simulink library "Susp_Components"  (R2026a)
settings: Solver=VariableStepAuto
undefined symbols (not defined in the file): Arm_to_Axle, clr_conn_links, clr_conn_rod, clr_link, clr_uaf, hp_in_f_ua, hp_out_f_ua, hp_shock_bot, hp_shock_botL, hp_shock_top, hp_shock_topL, hp_steerlink_out, hp_steerlink_outL, hp_upr_axle, hp_upr_axleL, hp_upr_drag, hp_upr_dragL, hp_wattsl_body, hp_wattsl_pivot, hp_wattsp_axle, hp_wattsu_body, hp_wattsu_pivot, hp_whl_ctr, hp_whl_ctrL, opc_conn_links, opc_conn_rod, opc_link, opc_uaf, radius_link, radius_uaf, size_conn_links, size_conn_rod, Susp, uaf_mass, upr_mass, Visual, wattsl_mass, wattsp_mass, wattsu_mass, X, Y, Z
libraries: sm_lib x32, Suspension_Utilities x10, Linkage_Shock x4, nesl_utility x3, $bdroot x2, simulink_extras x1
(part 1 of 2)
Description:
  | Component of Simscape Vehicle Templates Library
  | 
  | Copyright 2018-2025 The MathWorks, Inc.
settings Model: Creator=mwalker  LastModifiedBy=smiller

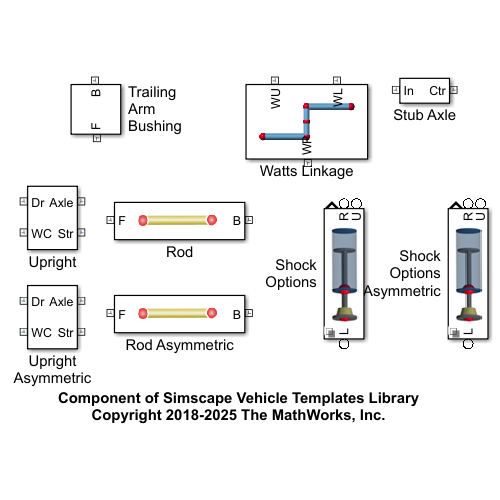
[thumbnail: Simulink's stored preview of the top-level diagram]
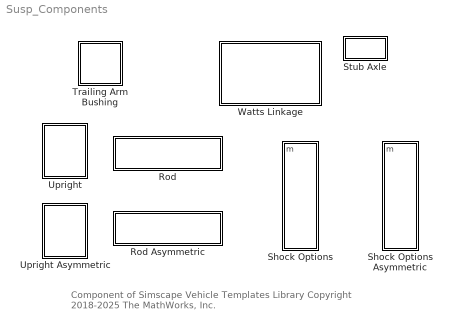
== system Susp_Components ==
  note: Component of Simscape Vehicle Templates Library
      | Copyright 2018-2025 The MathWorks, Inc.
  Rod : Subsystem  VariantControl=Steer  mask(Arm){popup_leftRight=Left, hp_in=hp_in_f_ua, hp_out=hp_out_f_ua, rod_mass=uaf_mass, clr_conn_rod=clr_conn_links, opc_conn_rod=opc_conn_links, size_conn_rod=size_conn_links, clr_rod=clr_uaf, opc_rod=opc_uaf, radius_rod=radius_uaf}
      mask prompts: popup_leftRight "Left/Right"; hp_in "HP B [xyz] (m)"; hp_out "HP F [xyz] (m)"; rod_mass "Mass (kg)"
      mask help: Rigid arm with two connection points.
      mask init:
      | if(popup_leftRight == 1)
      |     rhs_rod = 1;
      | elseif(popup_leftRight == 2)
      |     rhs_rod = -1;
      | end
      mask TypeOptions popup_leftRight: Left | Right
      mask TypeOptions rod_mass: Rod/Mass
      mask TypeOptions clr_conn_rod:
      | Vis
      | HP A/GraphicDiffuseColor | Vis
      | HP B/GraphicDiffuseColor
      mask TypeOptions opc_conn_rod:
      | Vis
      | HP A/GraphicOpacity | Vis
      | HP B/GraphicOpacity
      mask TypeOptions clr_rod: Rod/clr_solid
      mask TypeOptions opc_rod: Rod/opc_solid
      mask TypeOptions radius_rod: Rod/rad_solid
      mask DialogControl cont_rod Prompt: Rod
      mask DialogControl grp_rod Prompt: Rod
      mask DialogControl cont_vis_rod Prompt: Visualization
      mask DialogControl text_clr_rod Prompt: Color [RGB]
      mask DialogControl text_opc_rod Prompt: Opac. (0-1)
      mask DialogControl text_size_rod Prompt: Size (m)
      mask DialogControl text_conn_rod Prompt: Connections
      mask DialogControl text_rod_rod Prompt: Rod
      mask Display: image('sm_car_vehicle_linkage_link_IMAGE.png');
  Rod Asymmetric : Subsystem  VariantControl=Steer  mask(Arm){hp_in=hp_in_f_ua, hp_out=hp_out_f_ua, rod_mass=uaf_mass, clr_conn_rod=clr_conn_links, opc_conn_rod=opc_conn_links, size_conn_rod=size_conn_links, clr_rod=clr_uaf, opc_rod=opc_uaf, radius_rod=radius_uaf}
      mask prompts: hp_in "HP B [xyz] (m)"; hp_out "HP F [xyz] (m)"; rod_mass "Mass (kg)"
      mask help: Rigid arm with two connection points.
      mask TypeOptions rod_mass: Rod/Mass
      mask TypeOptions clr_conn_rod:
      | Vis
      | HP A/GraphicDiffuseColor | Vis
      | HP B/GraphicDiffuseColor
      mask TypeOptions opc_conn_rod:
      | Vis
      | HP A/GraphicOpacity | Vis
      | HP B/GraphicOpacity
      mask TypeOptions clr_rod: Rod/clr_solid
      mask TypeOptions opc_rod: Rod/opc_solid
      mask TypeOptions radius_rod: Rod/rad_solid
      mask DialogControl cont_rod Prompt: Rod
      mask DialogControl grp_rod Prompt: Rod
      mask DialogControl cont_vis_rod Prompt: Visualization
      mask DialogControl text_clr_rod Prompt: Color [RGB]
      mask DialogControl text_opc_rod Prompt: Opac. (0-1)
      mask DialogControl text_size_rod Prompt: Size (m)
      mask DialogControl text_conn_rod Prompt: Connections
      mask DialogControl text_rod_rod Prompt: Rod
      mask Display: image('sm_car_vehicle_linkage_link_IMAGE.png');
  Shock Options : Subsystem  Variant=on  VariantControlMode=label  VariantControl=ShockL  LabelModeActiveChoice=CylUpAttCtr  mask{popup_leftRight=Left, VariantLabel='CylUpAttCtr'}
      mask prompts: popup_leftRight "Left/Right"; VariantLabel "Variant Label"
      mask init:
      | curblk = gcb;
      | 
      | % Set variant for this block 
      | set_param(curblk,'LabelModeActiveChoice',VariantLabel);
      | 
      | if(popup_leftRight == 1)
      |     rhs_rod = 1;
      | elseif(popup_leftRight == 2)
      |     rhs_rod = -1;
      | end
      mask TypeOptions popup_leftRight: Left | Right
  Shock Options Asymmetric : Subsystem  Variant=on  VariantControlMode=label  VariantControl=ShockL  LabelModeActiveChoice=CylUpAttCtr  mask{hp_shock_top=hp_shock_topL, hp_shock_bot=hp_shock_botL, VariantLabel='CylUpAttCtr'}
      mask prompts: hp_shock_top "Spring Top [xyz] (m)"; hp_shock_bot "Spring Bottom [xyz] (m)"; VariantLabel "Variant Label"
      mask init:
      | curblk = gcb;
      | 
      | % Set variant for this block 
      | set_param(curblk,'LabelModeActiveChoice',VariantLabel);
  Stub Axle : Subsystem  mask{popup_leftRight=Left, stub_axle_len=Susp.AxleTA4Watts.Axle.xAxle.Value, stub_axle_mass=Susp.AxleTA4Watts.StubAxle.m.Value, clr_stub_axle=Visual.Axle.clr, opc_stub_axle=Visual.part.opc, rad_stub_axle=Visual.Axle.rad}
      mask prompts: popup_leftRight "Left/Right"; stub_axle_len "Stub Axle Length (m)"; stub_axle_mass "Stub Axle Mass (kg)"; clr_stub_axle "Color [RGB]"; opc_stub_axle "Opacity (0-1)"; rad_stub_axle "Stub Axle Radius (m)"
      mask init:
      | if(popup_leftRight == 1)
      |     rhs_rod = 1;
      | elseif(popup_leftRight == 2)
      |     rhs_rod = -1;
      | end
      mask TypeOptions popup_leftRight: Left | Right
      mask TypeOptions stub_axle_mass: Axle/Mass
      mask TypeOptions clr_stub_axle: Axle/GraphicDiffuseColor
      mask TypeOptions opc_stub_axle: Axle/GraphicOpacity
      mask TypeOptions rad_stub_axle: Axle/CylinderRadius
      mask DialogControl cont_vis Prompt: Visualization
  Trailing Arm Bushing : Subsystem  mask{Arm_to_Axle=Arm_to_Axle}
      mask prompts: Arm_to_Axle "Arm to Axle (structure)"
  Upright : Subsystem  mask(Upright, Three Connections){popup_leftRight=Left, clr_conn_rod=Visual.hp.clr, opc_conn_rod=Visual.hp.opc, size_conn_rod=Visual.hp.rad, clr_upr=Visual.Upright.clr, opc_upr=Visual.part.opc, rad_upr=Visual.Upright.rad}
      mask prompts: popup_leftRight "Left/Right"; clr_conn_rod "Connections Color [R G B] (0-1)"; opc_conn_rod "Connections Opacity (0-1)"; size_conn_rod "Connections Radius (m)"; clr_upr "Link Color [R G B] (0-1)"; opc_upr "Link Opacity (0-1)"; rad_upr "Link Radius (0-1)"
      mask help: Models an upright with connections to the axle along the kingpin axis (Axle), wheel center (WC), drag link (Dr), and steering link (Str).
      mask init:
      | if(popup_leftRight == 1)
      |     rhs_upr = 1;
      | elseif(popup_leftRight == 2)
      |     rhs_upr = -1;
      | end
      | rhs_hp = [1 rhs_upr 1];
      mask TypeOptions popup_leftRight: Left | Right
      mask DialogControl cont_vis Prompt: Visualization
  Upright Asymmetric : Subsystem  mask(Upright, Three Connections){hp_upr_axle=hp_upr_axleL, hp_whl_ctr=hp_whl_ctrL, hp_upr_drag=hp_upr_dragL, hp_steerlink_out=hp_steerlink_outL, clr_conn_rod=Visual.hp.clr, opc_conn_rod=Visual.hp.opc, size_conn_rod=Visual.hp.rad, clr_upr=Visual.Upright.clr, opc_upr=Visual.part.opc, rad_upr=Visual.Upright.rad}
      mask prompts: hp_upr_axle "Hardpoint Upright Axle [xyz] (m)"; hp_whl_ctr "Hardpoint Wheel Center [xyz] (m)"; hp_upr_drag "Hardpoint Drag Link [xyz] (m)"; hp_steerlink_out "Hardpoint Steer Link  [xyz] (m)"; clr_conn_rod "Connections Color [R G B] (0-1)"; opc_conn_rod "Connections Opacity (0-1)"; size_conn_rod "Connections Radius (m)"; clr_upr "Link Color [R G B] (0-1)"; opc_upr "Link Opacity (0-1)"; rad_upr "Link Radius (0-1)"
      mask help: Models an upright with connections to the axle along the kingpin axis (Axle), wheel center (WC), drag link (Dr), and steering link (Str).
      mask TypeOptions hp_upr_axle: Drag/hp_b | Steer/hp_b | Upright/hp_b
      mask TypeOptions hp_whl_ctr: Upright/hp_f
      mask TypeOptions hp_upr_drag: Drag/hp_f
      mask TypeOptions hp_steerlink_out: Steer/hp_f
      mask DialogControl cont_vis Prompt: Visualization
  Watts Linkage : Subsystem  mask(Watts Linkage){hp_wattsu_body=hp_wattsu_body, hp_wattsl_body=hp_wattsl_body, hp_wattsu_pivot=hp_wattsu_pivot, hp_wattsl_pivot=hp_wattsl_pivot, hp_wattsp_axle=hp_wattsp_axle, wattsu_mass=wattsu_mass, wattsl_mass=wattsl_mass, wattsp_mass=wattsp_mass, clr_conn_rod=clr_conn_rod, opc_conn_rod=opc_conn_rod, size_conn_rod=size_conn_rod, clr_link=clr_link, opc_link=opc_link, radius_link=radius_link}
      mask prompts: hp_wattsu_body "Watts Link Upper Body [xyz] (m)"; hp_wattsl_body "Watts Link Lower Body [xyz] (m)"; hp_wattsu_pivot "Watts Link Upper to Pivot [xyz] (m)"; hp_wattsl_pivot "Watts Link Lower to Pivot [xyz] (m)"; hp_wattsp_axle "Watts Link Pivot to Axle [xyz] (m)"; wattsu_mass "Watts Link Upper Mass (kg)"; wattsl_mass "Watts Link Lower Mass (kg)"; wattsp_mass "Watts Link Pivot Mass (kg)"
      mask help: Models a Watts linkage with upper, lower, and pivot links.
      mask TypeOptions hp_wattsu_body:
      | Watts Link
      | Upper/hp_in
      mask TypeOptions hp_wattsl_body:
      | Watts Link
      | Lower/hp_in
      mask TypeOptions hp_wattsu_pivot:
      | Watts Link
      | Pivot/hp_b | Watts Link
      | Upper/hp_out
      mask TypeOptions hp_wattsl_pivot:
      | Watts Link
      | Lower/hp_out | Watts Link
      | Pivot/hp_f
      mask TypeOptions hp_wattsp_axle:
      | Watts Link
      | Pivot/hp_piv
      mask TypeOptions wattsu_mass:
      | Watts Link
      | Upper/rod_mass
      mask TypeOptions wattsl_mass:
      | Watts Link
      | Lower/rod_mass
      mask TypeOptions wattsp_mass:
      | Watts Link
      | Pivot/rod_mass
      mask TypeOptions clr_conn_rod:
      | Watts Link
      | Lower/clr_conn_rod | Watts Link
      | Pivot/clr_conn_rod | Watts Link
      | Upper/clr_conn_rod
      mask TypeOptions opc_conn_rod:
      | Watts Link
      | Lower/opc_conn_rod | Watts Link
      | Pivot/opc_conn_rod | Watts Link
      | Upper/opc_conn_rod
      mask TypeOptions size_conn_rod:
      | Watts Link
      | Lower/size_conn_rod | Watts Link
      | Pivot/size_conn_rod | Watts Link
      | Upper/size_conn_rod
      mask TypeOptions clr_link:
      | Watts Link
      | Lower/clr_rod | Watts Link
      | Pivot/clr_rod | Watts Link
      | Upper/clr_rod
      mask TypeOptions opc_link:
      | Watts Link
      | Lower/opc_rod | Watts Link
      | Pivot/opc_rod | Watts Link
      | Upper/opc_rod
      mask TypeOptions radius_link:
      | Watts Link
      | Lower/radius_rod | Watts Link
      | Pivot/radius_rod | Watts Link
      | Upper/radius_rod
      mask DialogControl cont_hp Prompt: Hardpoints
      mask DialogControl cont_parts Prompt: Parts
      mask DialogControl cont_parts_vis Prompt: Visualization
      mask DialogControl text_vis_clr Prompt: Color [RGB]
      mask DialogControl text_vis_opc Prompt: Opac. (0-1)
      mask DialogControl text_vis_size Prompt: Size (m)
      mask DialogControl text_vis_conn Prompt: Connections
      mask DialogControl text_vis_links Prompt: Links
      mask Display: image('sm_car_vehicle_susp_wattslinkage_image.png');

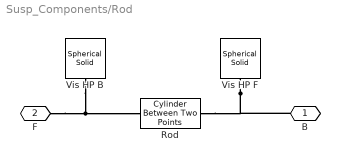
== system Susp_Components/Rod ==
  Rod : Suspension_Utilities/Cylinder Between Two Points  hp_b=hp_in.*[1 rhs_rod 1]  hp_f=hp_out.*[1 rhs_rod 1]  Mass=rod_mass  clr_solid=clr_rod  opc_solid=opc_rod  rad_solid=radius_rod
  Vis HP B : sm_lib/Body Elements/Spherical Solid  SphereRadius=size_conn_rod  SphereRadiusUnits=m  ExportEntireGeometry=off  InertiaType=CalculateFromGeometry  BasedOnType=Density  Density=0  DensityUnits=kg/m^3  Mass=1  MassUnits=kg  CenterOfMass=[0 0 0]  CenterOfMassUnits=m  MomentsOfInertia=[1 1 1]  MomentsOfInertiaUnits=kg*m^2  ProductsOfInertia=[0 0 0]  ProductsOfInertiaUnits=kg*m^2  GraphicType=FromGeometry  MarkerShape=Sphere  MarkerSize=10  GraphicVisPropType=SimpleVisualProperties  GraphicDiffuseColor=clr_conn_rod  GraphicOpacity=opc_conn_rod  GraphicSpecularColor=[0.5 0.5 0.5 1.0]  GraphicAmbientColor=[0.15 0.15 0.15 1.0]  GraphicEmissiveColor=[0.0 0.0 0.0 1.0]  GraphicShininess=75  DoExposeReferenceFrame=on  SerializedFrames=<Frames/>
  Vis HP F : sm_lib/Body Elements/Spherical Solid  SphereRadius=size_conn_rod  SphereRadiusUnits=m  ExportEntireGeometry=off  InertiaType=CalculateFromGeometry  BasedOnType=Density  Density=0  DensityUnits=kg/m^3  Mass=1  MassUnits=kg  CenterOfMass=[0 0 0]  CenterOfMassUnits=m  MomentsOfInertia=[1 1 1]  MomentsOfInertiaUnits=kg*m^2  ProductsOfInertia=[0 0 0]  ProductsOfInertiaUnits=kg*m^2  GraphicType=FromGeometry  MarkerShape=Sphere  MarkerSize=10  GraphicVisPropType=SimpleVisualProperties  GraphicDiffuseColor=clr_conn_rod  GraphicOpacity=opc_conn_rod  GraphicSpecularColor=[0.5 0.5 0.5 1.0]  GraphicAmbientColor=[0.15 0.15 0.15 1.0]  GraphicEmissiveColor=[0.0 0.0 0.0 1.0]  GraphicShininess=75  DoExposeReferenceFrame=on  SerializedFrames=<Frames/>
  B : PMIOPort  Side=Right
  F : PMIOPort  Port=2  Side=Left
  connections:
  Vis HP F/RConn1 -- B/RConn1 -- Rod/LConn1
  F/RConn1 -- Rod/RConn1 -- Vis HP B/RConn1

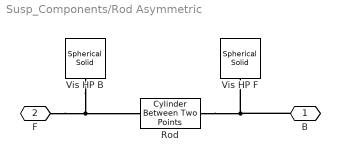
== system Susp_Components/Rod Asymmetric ==
  Rod : Suspension_Utilities/Cylinder Between Two Points  hp_b=hp_in  hp_f=hp_out  Mass=rod_mass  clr_solid=clr_rod  opc_solid=opc_rod  rad_solid=radius_rod
  Vis HP B : sm_lib/Body Elements/Spherical Solid  SphereRadius=size_conn_rod  SphereRadiusUnits=m  ExportEntireGeometry=off  InertiaType=CalculateFromGeometry  BasedOnType=Density  Density=0  DensityUnits=kg/m^3  Mass=1  MassUnits=kg  CenterOfMass=[0 0 0]  CenterOfMassUnits=m  MomentsOfInertia=[1 1 1]  MomentsOfInertiaUnits=kg*m^2  ProductsOfInertia=[0 0 0]  ProductsOfInertiaUnits=kg*m^2  GraphicType=FromGeometry  MarkerShape=Sphere  MarkerSize=10  GraphicVisPropType=SimpleVisualProperties  GraphicDiffuseColor=clr_conn_rod  GraphicOpacity=opc_conn_rod  GraphicSpecularColor=[0.5 0.5 0.5 1.0]  GraphicAmbientColor=[0.15 0.15 0.15 1.0]  GraphicEmissiveColor=[0.0 0.0 0.0 1.0]  GraphicShininess=75  DoExposeReferenceFrame=on  SerializedFrames=<Frames/>
  Vis HP F : sm_lib/Body Elements/Spherical Solid  SphereRadius=size_conn_rod  SphereRadiusUnits=m  ExportEntireGeometry=off  InertiaType=CalculateFromGeometry  BasedOnType=Density  Density=0  DensityUnits=kg/m^3  Mass=1  MassUnits=kg  CenterOfMass=[0 0 0]  CenterOfMassUnits=m  MomentsOfInertia=[1 1 1]  MomentsOfInertiaUnits=kg*m^2  ProductsOfInertia=[0 0 0]  ProductsOfInertiaUnits=kg*m^2  GraphicType=FromGeometry  MarkerShape=Sphere  MarkerSize=10  GraphicVisPropType=SimpleVisualProperties  GraphicDiffuseColor=clr_conn_rod  GraphicOpacity=opc_conn_rod  GraphicSpecularColor=[0.5 0.5 0.5 1.0]  GraphicAmbientColor=[0.15 0.15 0.15 1.0]  GraphicEmissiveColor=[0.0 0.0 0.0 1.0]  GraphicShininess=75  DoExposeReferenceFrame=on  SerializedFrames=<Frames/>
  B : PMIOPort  Side=Right
  F : PMIOPort  Port=2  Side=Left
  connections:
  Vis HP B/RConn1 -- Rod/RConn1 -- F/RConn1
  Rod/LConn1 -- B/RConn1 -- Vis HP F/RConn1

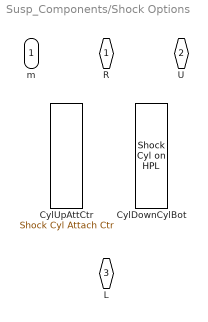
== system Susp_Components/Shock Options ==
  CylDownCylBot : Linkage_Shock/Shock Cyl on HPL  VariantControl=CylDownCylBot  shock_pist_mass=piston_mass  shock_cyl_mass=cyl_mass  hp_spr_top=hp_shock_top.*[1 rhs_rod 1]  hp_spr_bot=hp_shock_bot.*[1 rhs_rod 1]  up_lim_bumpstop=shock_xmax  low_lim_bumpstop=shock_xmin  clr_conn_shock=Visual.hp.clr  opc_conn_shock=Visual.hp.opc  size_conn_shock=Visual.hp.rad  clr_shock_cyl=Visual.clr.blue  opc_shock_cyl=Visual.part.opc  radius_shock_cyl=0.05  clr_shock_piston=Visual.clr.gray  opc_shock_piston=Visual.part.opc  clr_shock_bumpstop=Visual.clr.yellowpale  opc_shock_bumpstop=Visual.part.opc  deadvol_len_shock_cyl=Visual.Shock.dead_length  piston_len_shock=Visual.Shock.piston.len  cyl_cap_len_shock=Visual.Shock.cap.len  bumpstop_len_shock=Visual.Shock.bumpstop.len
  CylUpAttCtr : Linkage_Shock/Shock Cyl Attach Ctr  VariantControl=CylUpAttCtr  shock_pist_mass=piston_mass  shock_cyl_mass=cyl_mass  hp_spr_top=hp_shock_top.*[1 rhs_rod 1]  hp_spr_bot=hp_shock_bot.*[1 rhs_rod 1]  up_lim_bumpstop=shock_xmax  low_lim_bumpstop=shock_xmin  clr_conn_shock=Visual.hp.clr  opc_conn_shock=Visual.hp.opc  size_conn_shock=Visual.hp.rad  clr_shock_cyl=Visual.clr.blue  opc_shock_cyl=Visual.part.opc  radius_shock_cyl=0.05  clr_shock_piston=Visual.clr.gray  opc_shock_piston=Visual.part.opc  clr_shock_bumpstop=Visual.clr.yellowpale  opc_shock_bumpstop=Visual.part.opc  deadvol_len_shock_cyl=Visual.Shock.dead_length  piston_len_shock=Visual.Shock.piston.len  cyl_cap_len_shock=Visual.Shock.cap.len  bumpstop_len_shock=Visual.Shock.bumpstop.len
  R : PMIOPort  Side=Right
  U : PMIOPort  Port=2  Side=Right
  L : PMIOPort  Port=3  Side=Left
  m : Outport

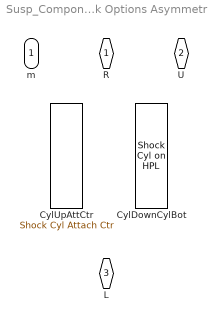
== system Susp_Components/Shock Options Asymmetric ==
  CylDownCylBot : Linkage_Shock/Shock Cyl on HPL  VariantControl=CylDownCylBot  shock_pist_mass=piston_mass  shock_cyl_mass=cyl_mass  hp_spr_top=hp_shock_top  hp_spr_bot=hp_shock_bot  up_lim_bumpstop=shock_xmax  low_lim_bumpstop=shock_xmin  clr_conn_shock=Visual.hp.clr  opc_conn_shock=Visual.hp.opc  size_conn_shock=Visual.hp.rad  clr_shock_cyl=Visual.clr.blue  opc_shock_cyl=Visual.part.opc  radius_shock_cyl=0.05  clr_shock_piston=Visual.clr.gray  opc_shock_piston=Visual.part.opc  clr_shock_bumpstop=Visual.clr.yellowpale  opc_shock_bumpstop=Visual.part.opc  deadvol_len_shock_cyl=Visual.Shock.dead_length  piston_len_shock=Visual.Shock.piston.len  cyl_cap_len_shock=Visual.Shock.cap.len  bumpstop_len_shock=Visual.Shock.bumpstop.len
  CylUpAttCtr : Linkage_Shock/Shock Cyl Attach Ctr  VariantControl=CylUpAttCtr  shock_pist_mass=piston_mass  shock_cyl_mass=cyl_mass  hp_spr_top=hp_shock_top  hp_spr_bot=hp_shock_bot  up_lim_bumpstop=shock_xmax  low_lim_bumpstop=shock_xmin  clr_conn_shock=Visual.hp.clr  opc_conn_shock=Visual.hp.opc  size_conn_shock=Visual.hp.rad  clr_shock_cyl=Visual.clr.blue  opc_shock_cyl=Visual.part.opc  radius_shock_cyl=0.05  clr_shock_piston=Visual.clr.gray  opc_shock_piston=Visual.part.opc  clr_shock_bumpstop=Visual.clr.yellowpale  opc_shock_bumpstop=Visual.part.opc  deadvol_len_shock_cyl=Visual.Shock.dead_length  piston_len_shock=Visual.Shock.piston.len  cyl_cap_len_shock=Visual.Shock.cap.len  bumpstop_len_shock=Visual.Shock.bumpstop.len
  R : PMIOPort  Side=Right
  U : PMIOPort  Port=2  Side=Right
  L : PMIOPort  Port=3  Side=Left
  m : Outport

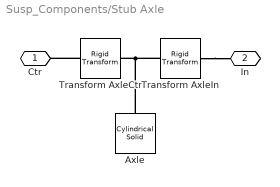
== system Susp_Components/Stub Axle ==
  Axle : sm_lib/Body Elements/Cylindrical Solid  CylinderRadius=rad_stub_axle  CylinderRadiusUnits=m  CylinderLength=stub_axle_len  CylinderLengthUnits=m  ExportEntireGeometry=off  InertiaType=CalculateFromGeometry  BasedOnType=Mass  Density=7000  DensityUnits=kg/m^3  Mass=stub_axle_mass  MassUnits=kg  CenterOfMass=[0 0 0]  CenterOfMassUnits=m  MomentsOfInertia=[1 1 1]  MomentsOfInertiaUnits=kg*m^2  ProductsOfInertia=[0 0 0]  ProductsOfInertiaUnits=kg*m^2  GraphicType=FromGeometry  MarkerShape=Sphere  MarkerSize=10  GraphicVisPropType=SimpleVisualProperties  GraphicDiffuseColor=clr_stub_axle  GraphicOpacity=opc_stub_axle  GraphicSpecularColor=[0.5 0.5 0.5 1.0]  GraphicAmbientColor=[0.15 0.15 0.15 1.0]  GraphicEmissiveColor=[0.0 0.0 0.0 1.0]  GraphicShininess=75  DoExposeReferenceFrame=on  SerializedFrames=<Frames/>
  Transform AxleCtr : sm_lib/Frames and Transforms/Rigid Transform  RotationMethod=None  FollAlignAxisA=+X  BaseAlignAxisA=+Y  FollAlignAxisB=+Y  BaseAlignAxisB=+Z  RotationStandardAxis=+Z  RotationAngle=0  RotationAngleUnits=deg  RotationArbitraryAxis=[0 0 1]  RotationSequenceAxes=FollowerAxes  RotationSequence=XYX  RotationSequenceAngles=[0 0 0]  RotationSequenceAnglesUnits=deg  RotationMatrix=[1 0 0; 0 1 0; 0 0 1]  Quaternion=[1 0 0 0]  TranslationMethod=StandardAxis  TranslationCartesianOffset=[0 0 0]  TranslationCartesianOffsetUnits=m  TranslationStandardAxis=-Z  TranslationStandardOffset=rhs_rod*stub_axle_len/2  TranslationStandardOffsetUnits=m  TranslationROffset=0  TranslationROffsetUnits=m  TranslationThetaOffset=0  TranslationThetaOffsetUnits=deg  TranslationZOffset=0  TranslationZOffsetUnits=m
  Transform AxleIn : sm_lib/Frames and Transforms/Rigid Transform  RotationMethod=None  FollAlignAxisA=+X  BaseAlignAxisA=+Y  FollAlignAxisB=+Y  BaseAlignAxisB=+Z  RotationStandardAxis=+Z  RotationAngle=0  RotationAngleUnits=deg  RotationArbitraryAxis=[0 0 1]  RotationSequenceAxes=FollowerAxes  RotationSequence=XYX  RotationSequenceAngles=[0 0 0]  RotationSequenceAnglesUnits=deg  RotationMatrix=[1 0 0; 0 1 0; 0 0 1]  Quaternion=[1 0 0 0]  TranslationMethod=StandardAxis  TranslationCartesianOffset=[0 0 0]  TranslationCartesianOffsetUnits=m  TranslationStandardAxis=-Z  TranslationStandardOffset=rhs_rod*stub_axle_len/2  TranslationStandardOffsetUnits=m  TranslationROffset=0  TranslationROffsetUnits=m  TranslationThetaOffset=0  TranslationThetaOffsetUnits=deg  TranslationZOffset=0  TranslationZOffsetUnits=m
  Ctr : PMIOPort  Side=Left
  In : PMIOPort  Port=2  Side=Right
  connections:
  Transform AxleIn/RConn1 -- In/RConn1
  Transform AxleCtr/LConn1 -- Ctr/RConn1
  Transform AxleIn/LConn1 -- Transform AxleCtr/RConn1 -- Axle/RConn1

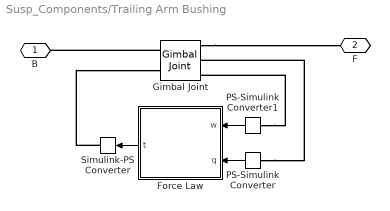
== system Susp_Components/Trailing Arm Bushing ==
  Force Law : Subsystem  mask{nLinear=Arm_to_Axle.Damping.nLinear.Value, nCubic=Arm_to_Axle.Damping.nCubic.Value, qStiffness=Arm_to_Axle.Stiffness.q.Value, trqStiffness=Arm_to_Axle.Stiffness.trq.Value, wFriction=Arm_to_Axle.Friction.w.Value, trqFriction=Arm_to_Axle.Friction.trq.Value}
      mask prompts: nLinear "Linear Gain"; nCubic "Cubic Gain"; qStiffness "Angle (rad)"; trqStiffness "Torque (N*m)"; wFriction "Rotational Velocity (rad/s)"; trqFriction "Torque (N*m)"
      mask TypeOptions nLinear: Gain Linear Term/Gain
      mask TypeOptions nCubic: Gain Exp Term/Gain
      mask TypeOptions qStiffness: Torsional Stiffness/BreakpointsForDimension1
      mask TypeOptions trqStiffness: Torsional Stiffness/Table
      mask TypeOptions wFriction: Friction/BreakpointsForDimension1
      mask TypeOptions trqFriction: Friction/Table
      mask DialogControl grpStiffness Prompt: Stiffness
      mask DialogControl grpFriction Prompt: Friction
      mask DialogControl grpDamping Prompt: Damping
  Gimbal Joint : sm_lib/Joints/Gimbal Joint  JointMode=Normal  CompositeWrenchDir=FollowerOnBase  CompositeWrenchFrame=BaseFrame  SenseConstraintForce=off  SenseConstraintTorque=off  SenseTotalForce=off  SenseTotalTorque=off  RxPositionTargetSpecify=on  RxPositionTargetPriority=Low  RxPositionTargetValue=0  RxPositionTargetValueUnits=deg  RxVelocityTargetSpecify=off  RxVelocityTargetPriority=High  RxVelocityTargetValue=0  RxVelocityTargetValueUnits=deg/s  RxEquilibriumPosition=0  RxEquilibriumPositionUnits=deg  RxSpringStiffness=0  RxSpringStiffnessUnits=N*m/deg  RxDampingCoefficient=0  RxDampingCoefficientUnits=N*m/(deg/s)  RxLowerLimitSpecify=off  RxLowerLimitBound=-90  RxLowerLimitBoundUnits=deg  RxLowerLimitStiffness=1e4  RxLowerLimitStiffnessUnits=N*m/deg  RxLowerLimitDamping=10  RxLowerLimitDampingUnits=N*m/(deg/s)  RxLowerLimitTransitionRegionWidth=0.1  RxLowerLimitTransitionRegionWidthUnits=deg  RxUpperLimitSpecify=off  RxUpperLimitBound=90  RxUpperLimitBoundUnits=deg  RxUpperLimitStiffness=1e4  RxUpperLimitStiffnessUnits=N*m/deg  RxUpperLimitDamping=10  RxUpperLimitDampingUnits=N*m/(deg/s)  RxUpperLimitTransitionRegionWidth=0.1  RxUpperLimitTransitionRegionWidthUnits=deg  RxTorqueActuationMode=NoTorque  RxMotionActuationMode=ComputedMotion  RxSensePosition=off  RxSenseVelocity=off  RxSenseAcceleration=off  RxSenseTorqueForce=off  RxSenseLowerLimitTorqueForce=off  RxSenseUpperLimitTorqueForce=off  RyPositionTargetSpecify=on  RyPositionTargetPriority=Low  RyPositionTargetValue=0  RyPositionTargetValueUnits=deg  RyVelocityTargetSpecify=off  RyVelocityTargetPriority=High  RyVelocityTargetValue=0  RyVelocityTargetValueUnits=deg/s  RyEquilibriumPosition=0  RyEquilibriumPositionUnits=deg  RySpringStiffness=0  RySpringStiffnessUnits=N*m/deg  RyDampingCoefficient=0  RyDampingCoefficientUnits=N*m/(deg/s)  RyLowerLimitSpecify=off  RyLowerLimitBound=-90  RyLowerLimitBoundUnits=deg  RyLowerLimitStiffness=1e4  RyLowerLimitStiffnessUnits=N*m/deg  RyLowerLimitDamping=10  RyLowerLimitDampingUnits=N*m/(deg/s)  RyLowerLimitTransitionRegionWidth=0.1  RyLowerLimitTransitionRegionWidthUnits=deg  RyUpperLimitSpecify=off  RyUpperLimitBound=90  RyUpperLimitBoundUnits=deg  RyUpperLimitStiffness=1e4  RyUpperLimitStiffnessUnits=N*m/deg  RyUpperLimitDamping=10  RyUpperLimitDampingUnits=N*m/(deg/s)  RyUpperLimitTransitionRegionWidth=0.1  RyUpperLimitTransitionRegionWidthUnits=deg  RyTorqueActuationMode=InputTorque  RyMotionActuationMode=ComputedMotion  RySensePosition=on  RySenseVelocity=on  RySenseAcceleration=off  RySenseTorqueForce=off  RySenseLowerLimitTorqueForce=off  RySenseUpperLimitTorqueForce=off  RzPositionTargetSpecify=off  RzPositionTargetPriority=High  RzPositionTargetValue=0  RzPositionTargetValueUnits=deg  RzVelocityTargetSpecify=off  RzVelocityTargetPriority=High  RzVelocityTargetValue=0  RzVelocityTargetValueUnits=deg/s  RzEquilibriumPosition=0  RzEquilibriumPositionUnits=deg  RzSpringStiffness=0  RzSpringStiffnessUnits=N*m/deg  RzDampingCoefficient=0  RzDampingCoefficientUnits=N*m/(deg/s)  RzLowerLimitSpecify=off  RzLowerLimitBound=-90  RzLowerLimitBoundUnits=deg  RzLowerLimitStiffness=1e4  RzLowerLimitStiffnessUnits=N*m/deg  RzLowerLimitDamping=10  RzLowerLimitDampingUnits=N*m/(deg/s)  RzLowerLimitTransitionRegionWidth=0.1  RzLowerLimitTransitionRegionWidthUnits=deg  RzUpperLimitSpecify=off  RzUpperLimitBound=90  RzUpperLimitBoundUnits=deg  RzUpperLimitStiffness=1e4  RzUpperLimitStiffnessUnits=N*m/deg  RzUpperLimitDamping=10  RzUpperLimitDampingUnits=N*m/(deg/s)  RzUpperLimitTransitionRegionWidth=0.1  RzUpperLimitTransitionRegionWidthUnits=deg  RzTorqueActuationMode=NoTorque  RzMotionActuationMode=ComputedMotion  RzSensePosition=off  RzSenseVelocity=off  RzSenseAcceleration=off  RzSenseTorqueForce=off  RzSenseLowerLimitTorqueForce=off  RzSenseUpperLimitTorqueForce=off
  PS-Simulink Converter : nesl_utility/PS-Simulink Converter  PhysicalDomain=network_engine_domain  SubClassName=ps_output  LeftPortType=input  RightPortType=output  PseudoPeriodic=off  Frequencies=[]  VectorFormat=inherit  Unit=inherit  AffineConversion=off
  PS-Simulink Converter1 : nesl_utility/PS-Simulink Converter  PhysicalDomain=network_engine_domain  SubClassName=ps_output  LeftPortType=input  RightPortType=output  PseudoPeriodic=off  Frequencies=[]  VectorFormat=inherit  Unit=inherit  AffineConversion=off
  Simulink-PS Converter : nesl_utility/Simulink-PS Converter  PhysicalDomain=network_engine_domain  SubClassName=ps_input  LeftPortType=input  RightPortType=output  PseudoPeriodic=off  Frequencies=[]  NoiseDistribution=none  NoiseParameters=[]  Unit=1  AffineConversion=off  FilteringAndDerivatives=provide  SimscapeFilterOrder=1  InputFilterTimeConstant=0.001  UdotUserProvided=0
  B : PMIOPort  Side=Left
  F : PMIOPort  Port=2  Side=Right
  wires:
  Force Law/1(t) -> Simulink-PS Converter/1
  PS-Simulink Converter1/1 -> Force Law/1(w)
  PS-Simulink Converter/1 -> Force Law/2(q)
  connections:
  PS-Simulink Converter/LConn1 -- Gimbal Joint/RConn2
  PS-Simulink Converter1/LConn1 -- Gimbal Joint/RConn3
  Simulink-PS Converter/RConn1 -- Gimbal Joint/LConn2
  Gimbal Joint/LConn1 -- B/RConn1
  Gimbal Joint/RConn1 -- F/RConn1

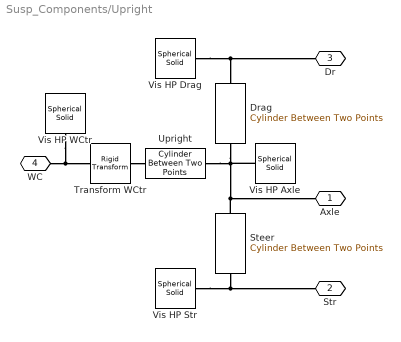
== system Susp_Components/Upright ==
  Drag : Suspension_Utilities/Cylinder Between Two Points  hp_b=hp_upr_axle.*rhs_hp  hp_f=hp_upr_drag.*rhs_hp  Mass=upr_mass/3  clr_solid=clr_upr  opc_solid=opc_upr  rad_solid=radius_upr
  Steer : Suspension_Utilities/Cylinder Between Two Points  hp_b=hp_upr_axle.*rhs_hp  hp_f=hp_steerlink_out.*rhs_hp  Mass=upr_mass/3  clr_solid=clr_upr  opc_solid=opc_upr  rad_solid=radius_upr
  Transform WCtr : sm_lib/Frames and Transforms/Rigid Transform  RotationMethod=StandardAxis  FollAlignAxisA=+X  BaseAlignAxisA=+Y  FollAlignAxisB=+Y  BaseAlignAxisB=+Z  RotationStandardAxis=+X  RotationAngle=-90  RotationAngleUnits=deg  RotationArbitraryAxis=[0 0 1]  RotationSequenceAxes=FollowerAxes  RotationSequence=XYX  RotationSequenceAngles=[0 0 0]  RotationSequenceAnglesUnits=deg  RotationMatrix=[1 0 0;0 1 0;0 0 1]  Quaternion=[1 0 0 0]  TranslationMethod=None  TranslationCartesianOffset=[0 0 0]  TranslationCartesianOffsetUnits=m  TranslationStandardAxis=+Z  TranslationStandardOffset=0  TranslationStandardOffsetUnits=m  TranslationROffset=0  TranslationROffsetUnits=m  TranslationThetaOffset=0  TranslationThetaOffsetUnits=deg  TranslationZOffset=0  TranslationZOffsetUnits=m
  Upright : Suspension_Utilities/Cylinder Between Two Points  hp_b=hp_upr_axle.*rhs_hp  hp_f=hp_whl_ctr.*rhs_hp  Mass=upr_mass/3  clr_solid=clr_upr  opc_solid=opc_upr  rad_solid=radius_upr
  Vis HP WCtr : sm_lib/Body Elements/Spherical Solid  SphereRadius=size_conn_rod  SphereRadiusUnits=m  ExportEntireGeometry=off  InertiaType=CalculateFromGeometry  BasedOnType=Density  Density=0  DensityUnits=kg/m^3  Mass=1  MassUnits=kg  CenterOfMass=[0 0 0]  CenterOfMassUnits=m  MomentsOfInertia=[1 1 1]  MomentsOfInertiaUnits=kg*m^2  ProductsOfInertia=[0 0 0]  ProductsOfInertiaUnits=kg*m^2  GraphicType=FromGeometry  MarkerShape=Sphere  MarkerSize=10  GraphicVisPropType=SimpleVisualProperties  GraphicDiffuseColor=clr_conn_rod  GraphicOpacity=opc_conn_rod  GraphicSpecularColor=[0.5 0.5 0.5 1.0]  GraphicAmbientColor=[0.15 0.15 0.15 1.0]  GraphicEmissiveColor=[0.0 0.0 0.0 1.0]  GraphicShininess=75  DoExposeReferenceFrame=on  SerializedFrames=<Frames/>
  Vis HP Axle : sm_lib/Body Elements/Spherical Solid  SphereRadius=size_conn_rod  SphereRadiusUnits=m  ExportEntireGeometry=off  InertiaType=CalculateFromGeometry  BasedOnType=Density  Density=0  DensityUnits=kg/m^3  Mass=1  MassUnits=kg  CenterOfMass=[0 0 0]  CenterOfMassUnits=m  MomentsOfInertia=[1 1 1]  MomentsOfInertiaUnits=kg*m^2  ProductsOfInertia=[0 0 0]  ProductsOfInertiaUnits=kg*m^2  GraphicType=FromGeometry  MarkerShape=Sphere  MarkerSize=10  GraphicVisPropType=SimpleVisualProperties  GraphicDiffuseColor=clr_conn_rod  GraphicOpacity=opc_conn_rod  GraphicSpecularColor=[0.5 0.5 0.5 1.0]  GraphicAmbientColor=[0.15 0.15 0.15 1.0]  GraphicEmissiveColor=[0.0 0.0 0.0 1.0]  GraphicShininess=75  DoExposeReferenceFrame=on  SerializedFrames=<Frames/>
  Vis HP Drag : sm_lib/Body Elements/Spherical Solid  SphereRadius=size_conn_rod  SphereRadiusUnits=m  ExportEntireGeometry=off  InertiaType=CalculateFromGeometry  BasedOnType=Density  Density=0  DensityUnits=kg/m^3  Mass=1  MassUnits=kg  CenterOfMass=[0 0 0]  CenterOfMassUnits=m  MomentsOfInertia=[1 1 1]  MomentsOfInertiaUnits=kg*m^2  ProductsOfInertia=[0 0 0]  ProductsOfInertiaUnits=kg*m^2  GraphicType=FromGeometry  MarkerShape=Sphere  MarkerSize=10  GraphicVisPropType=SimpleVisualProperties  GraphicDiffuseColor=clr_conn_rod  GraphicOpacity=opc_conn_rod  GraphicSpecularColor=[0.5 0.5 0.5 1.0]  GraphicAmbientColor=[0.15 0.15 0.15 1.0]  GraphicEmissiveColor=[0.0 0.0 0.0 1.0]  GraphicShininess=75  DoExposeReferenceFrame=on  SerializedFrames=<Frames/>
  Vis HP Str : sm_lib/Body Elements/Spherical Solid  SphereRadius=size_conn_rod  SphereRadiusUnits=m  ExportEntireGeometry=off  InertiaType=CalculateFromGeometry  BasedOnType=Density  Density=0  DensityUnits=kg/m^3  Mass=1  MassUnits=kg  CenterOfMass=[0 0 0]  CenterOfMassUnits=m  MomentsOfInertia=[1 1 1]  MomentsOfInertiaUnits=kg*m^2  ProductsOfInertia=[0 0 0]  ProductsOfInertiaUnits=kg*m^2  GraphicType=FromGeometry  MarkerShape=Sphere  MarkerSize=10  GraphicVisPropType=SimpleVisualProperties  GraphicDiffuseColor=clr_conn_rod  GraphicOpacity=opc_conn_rod  GraphicSpecularColor=[0.5 0.5 0.5 1.0]  GraphicAmbientColor=[0.15 0.15 0.15 1.0]  GraphicEmissiveColor=[0.0 0.0 0.0 1.0]  GraphicShininess=75  DoExposeReferenceFrame=on  SerializedFrames=<Frames/>
  Axle : PMIOPort  Side=Right
  Str : PMIOPort  Port=2  Side=Right
  Dr : PMIOPort  Port=3  Side=Left
  WC : PMIOPort  Port=4  Side=Left
  connections:
  Transform WCtr/LConn1 -- Upright/RConn1
  Vis HP Str/RConn1 -- Str/RConn1 -- Steer/RConn1
  Upright/LConn1 -- Axle/RConn1 -- Steer/LConn1 -- Drag/LConn1 -- Vis HP Axle/RConn1
  WC/RConn1 -- Vis HP WCtr/RConn1 -- Transform WCtr/RConn1
  Vis HP Drag/RConn1 -- Drag/RConn1 -- Dr/RConn1

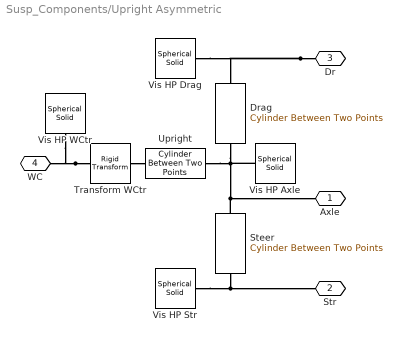
== system Susp_Components/Upright Asymmetric ==
  Drag : Suspension_Utilities/Cylinder Between Two Points  hp_b=hp_upr_axle  hp_f=hp_upr_drag  Mass=upr_mass/3  clr_solid=clr_upr  opc_solid=opc_upr  rad_solid=radius_upr
  Steer : Suspension_Utilities/Cylinder Between Two Points  hp_b=hp_upr_axle  hp_f=hp_steerlink_out  Mass=upr_mass/3  clr_solid=clr_upr  opc_solid=opc_upr  rad_solid=radius_upr
  Transform WCtr : sm_lib/Frames and Transforms/Rigid Transform  RotationMethod=StandardAxis  FollAlignAxisA=+X  BaseAlignAxisA=+Y  FollAlignAxisB=+Y  BaseAlignAxisB=+Z  RotationStandardAxis=+X  RotationAngle=-90  RotationAngleUnits=deg  RotationArbitraryAxis=[0 0 1]  RotationSequenceAxes=FollowerAxes  RotationSequence=XYX  RotationSequenceAngles=[0 0 0]  RotationSequenceAnglesUnits=deg  RotationMatrix=[1 0 0;0 1 0;0 0 1]  Quaternion=[1 0 0 0]  TranslationMethod=None  TranslationCartesianOffset=[0 0 0]  TranslationCartesianOffsetUnits=m  TranslationStandardAxis=+Z  TranslationStandardOffset=0  TranslationStandardOffsetUnits=m  TranslationROffset=0  TranslationROffsetUnits=m  TranslationThetaOffset=0  TranslationThetaOffsetUnits=deg  TranslationZOffset=0  TranslationZOffsetUnits=m
  Upright : Suspension_Utilities/Cylinder Between Two Points  hp_b=hp_upr_axle  hp_f=hp_whl_ctr  Mass=upr_mass/3  clr_solid=clr_upr  opc_solid=opc_upr  rad_solid=radius_upr
  Vis HP WCtr : sm_lib/Body Elements/Spherical Solid  SphereRadius=size_conn_rod  SphereRadiusUnits=m  ExportEntireGeometry=off  InertiaType=CalculateFromGeometry  BasedOnType=Density  Density=0  DensityUnits=kg/m^3  Mass=1  MassUnits=kg  CenterOfMass=[0 0 0]  CenterOfMassUnits=m  MomentsOfInertia=[1 1 1]  MomentsOfInertiaUnits=kg*m^2  ProductsOfInertia=[0 0 0]  ProductsOfInertiaUnits=kg*m^2  GraphicType=FromGeometry  MarkerShape=Sphere  MarkerSize=10  GraphicVisPropType=SimpleVisualProperties  GraphicDiffuseColor=clr_conn_rod  GraphicOpacity=opc_conn_rod  GraphicSpecularColor=[0.5 0.5 0.5 1.0]  GraphicAmbientColor=[0.15 0.15 0.15 1.0]  GraphicEmissiveColor=[0.0 0.0 0.0 1.0]  GraphicShininess=75  DoExposeReferenceFrame=on  SerializedFrames=<Frames/>
  Vis HP Axle : sm_lib/Body Elements/Spherical Solid  SphereRadius=size_conn_rod  SphereRadiusUnits=m  ExportEntireGeometry=off  InertiaType=CalculateFromGeometry  BasedOnType=Density  Density=0  DensityUnits=kg/m^3  Mass=1  MassUnits=kg  CenterOfMass=[0 0 0]  CenterOfMassUnits=m  MomentsOfInertia=[1 1 1]  MomentsOfInertiaUnits=kg*m^2  ProductsOfInertia=[0 0 0]  ProductsOfInertiaUnits=kg*m^2  GraphicType=FromGeometry  MarkerShape=Sphere  MarkerSize=10  GraphicVisPropType=SimpleVisualProperties  GraphicDiffuseColor=clr_conn_rod  GraphicOpacity=opc_conn_rod  GraphicSpecularColor=[0.5 0.5 0.5 1.0]  GraphicAmbientColor=[0.15 0.15 0.15 1.0]  GraphicEmissiveColor=[0.0 0.0 0.0 1.0]  GraphicShininess=75  DoExposeReferenceFrame=on  SerializedFrames=<Frames/>
  Vis HP Drag : sm_lib/Body Elements/Spherical Solid  SphereRadius=size_conn_rod  SphereRadiusUnits=m  ExportEntireGeometry=off  InertiaType=CalculateFromGeometry  BasedOnType=Density  Density=0  DensityUnits=kg/m^3  Mass=1  MassUnits=kg  CenterOfMass=[0 0 0]  CenterOfMassUnits=m  MomentsOfInertia=[1 1 1]  MomentsOfInertiaUnits=kg*m^2  ProductsOfInertia=[0 0 0]  ProductsOfInertiaUnits=kg*m^2  GraphicType=FromGeometry  MarkerShape=Sphere  MarkerSize=10  GraphicVisPropType=SimpleVisualProperties  GraphicDiffuseColor=clr_conn_rod  GraphicOpacity=opc_conn_rod  GraphicSpecularColor=[0.5 0.5 0.5 1.0]  GraphicAmbientColor=[0.15 0.15 0.15 1.0]  GraphicEmissiveColor=[0.0 0.0 0.0 1.0]  GraphicShininess=75  DoExposeReferenceFrame=on  SerializedFrames=<Frames/>
  Vis HP Str : sm_lib/Body Elements/Spherical Solid  SphereRadius=size_conn_rod  SphereRadiusUnits=m  ExportEntireGeometry=off  InertiaType=CalculateFromGeometry  BasedOnType=Density  Density=0  DensityUnits=kg/m^3  Mass=1  MassUnits=kg  CenterOfMass=[0 0 0]  CenterOfMassUnits=m  MomentsOfInertia=[1 1 1]  MomentsOfInertiaUnits=kg*m^2  ProductsOfInertia=[0 0 0]  ProductsOfInertiaUnits=kg*m^2  GraphicType=FromGeometry  MarkerShape=Sphere  MarkerSize=10  GraphicVisPropType=SimpleVisualProperties  GraphicDiffuseColor=clr_conn_rod  GraphicOpacity=opc_conn_rod  GraphicSpecularColor=[0.5 0.5 0.5 1.0]  GraphicAmbientColor=[0.15 0.15 0.15 1.0]  GraphicEmissiveColor=[0.0 0.0 0.0 1.0]  GraphicShininess=75  DoExposeReferenceFrame=on  SerializedFrames=<Frames/>
  Axle : PMIOPort  Side=Right
  Str : PMIOPort  Port=2  Side=Right
  Dr : PMIOPort  Port=3  Side=Left
  WC : PMIOPort  Port=4  Side=Left
  connections:
  Dr/RConn1 -- Drag/RConn1 -- Vis HP Drag/RConn1
  Transform WCtr/RConn1 -- Vis HP WCtr/RConn1 -- WC/RConn1
  Vis HP Axle/RConn1 -- Drag/LConn1 -- Steer/LConn1 -- Axle/RConn1 -- Upright/LConn1
  Steer/RConn1 -- Str/RConn1 -- Vis HP Str/RConn1
  Transform WCtr/LConn1 -- Upright/RConn1

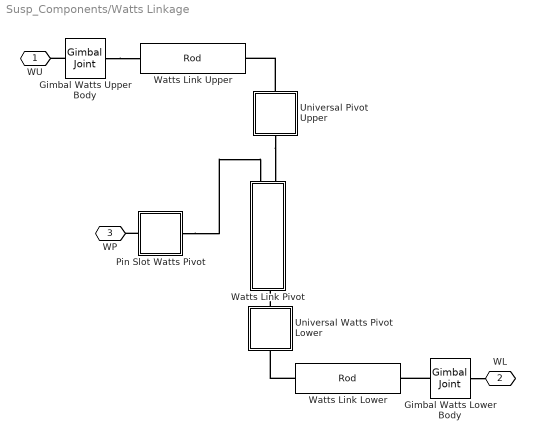
== system Susp_Components/Watts Linkage ==
  "Gimbal Watts Lower Body " : sm_lib/Joints/Gimbal Joint  JointMode=Normal  CompositeWrenchDir=FollowerOnBase  CompositeWrenchFrame=BaseFrame  SenseConstraintForce=off  SenseConstraintTorque=off  SenseTotalForce=off  SenseTotalTorque=off  RxPositionTargetSpecify=off  RxPositionTargetPriority=High  RxPositionTargetValue=0  RxPositionTargetValueUnits=deg  RxVelocityTargetSpecify=off  RxVelocityTargetPriority=High  RxVelocityTargetValue=0  RxVelocityTargetValueUnits=deg/s  RxEquilibriumPosition=0  RxEquilibriumPositionUnits=deg  RxSpringStiffness=0  RxSpringStiffnessUnits=N*m/deg  RxDampingCoefficient=0  RxDampingCoefficientUnits=N*m/(deg/s)  RxLowerLimitSpecify=off  RxLowerLimitBound=-90  RxLowerLimitBoundUnits=deg  RxLowerLimitStiffness=1e4  RxLowerLimitStiffnessUnits=N*m/deg  RxLowerLimitDamping=10  RxLowerLimitDampingUnits=N*m/(deg/s)  RxLowerLimitTransitionRegionWidth=0.1  RxLowerLimitTransitionRegionWidthUnits=deg  RxUpperLimitSpecify=off  RxUpperLimitBound=90  RxUpperLimitBoundUnits=deg  RxUpperLimitStiffness=1e4  RxUpperLimitStiffnessUnits=N*m/deg  RxUpperLimitDamping=10  RxUpperLimitDampingUnits=N*m/(deg/s)  RxUpperLimitTransitionRegionWidth=0.1  RxUpperLimitTransitionRegionWidthUnits=deg  RxTorqueActuationMode=NoTorque  RxMotionActuationMode=ComputedMotion  RxSensePosition=off  RxSenseVelocity=off  RxSenseAcceleration=off  RxSenseTorqueForce=off  RxSenseLowerLimitTorqueForce=off  RxSenseUpperLimitTorqueForce=off  RyPositionTargetSpecify=off  RyPositionTargetPriority=High  RyPositionTargetValue=0  RyPositionTargetValueUnits=deg  RyVelocityTargetSpecify=off  RyVelocityTargetPriority=High  RyVelocityTargetValue=0  RyVelocityTargetValueUnits=deg/s  RyEquilibriumPosition=0  RyEquilibriumPositionUnits=deg  RySpringStiffness=0  RySpringStiffnessUnits=N*m/deg  RyDampingCoefficient=0  RyDampingCoefficientUnits=N*m/(deg/s)  RyLowerLimitSpecify=off  RyLowerLimitBound=-90  RyLowerLimitBoundUnits=deg  RyLowerLimitStiffness=1e4  RyLowerLimitStiffnessUnits=N*m/deg  RyLowerLimitDamping=10  RyLowerLimitDampingUnits=N*m/(deg/s)  RyLowerLimitTransitionRegionWidth=0.1  RyLowerLimitTransitionRegionWidthUnits=deg  RyUpperLimitSpecify=off  RyUpperLimitBound=90  RyUpperLimitBoundUnits=deg  RyUpperLimitStiffness=1e4  RyUpperLimitStiffnessUnits=N*m/deg  RyUpperLimitDamping=10  RyUpperLimitDampingUnits=N*m/(deg/s)  RyUpperLimitTransitionRegionWidth=0.1  RyUpperLimitTransitionRegionWidthUnits=deg  RyTorqueActuationMode=NoTorque  RyMotionActuationMode=ComputedMotion  RySensePosition=off  RySenseVelocity=off  RySenseAcceleration=off  RySenseTorqueForce=off  RySenseLowerLimitTorqueForce=off  RySenseUpperLimitTorqueForce=off  RzPositionTargetSpecify=off  RzPositionTargetPriority=High  RzPositionTargetValue=0  RzPositionTargetValueUnits=deg  RzVelocityTargetSpecify=off  RzVelocityTargetPriority=High  RzVelocityTargetValue=0  RzVelocityTargetValueUnits=deg/s  RzEquilibriumPosition=0  RzEquilibriumPositionUnits=deg  RzSpringStiffness=0  RzSpringStiffnessUnits=N*m/deg  RzDampingCoefficient=0  RzDampingCoefficientUnits=N*m/(deg/s)  RzLowerLimitSpecify=off  RzLowerLimitBound=-90  RzLowerLimitBoundUnits=deg  RzLowerLimitStiffness=1e4  RzLowerLimitStiffnessUnits=N*m/deg  RzLowerLimitDamping=10  RzLowerLimitDampingUnits=N*m/(deg/s)  RzLowerLimitTransitionRegionWidth=0.1  RzLowerLimitTransitionRegionWidthUnits=deg  RzUpperLimitSpecify=off  RzUpperLimitBound=90  RzUpperLimitBoundUnits=deg  RzUpperLimitStiffness=1e4  RzUpperLimitStiffnessUnits=N*m/deg  RzUpperLimitDamping=10  RzUpperLimitDampingUnits=N*m/(deg/s)  RzUpperLimitTransitionRegionWidth=0.1  RzUpperLimitTransitionRegionWidthUnits=deg  RzTorqueActuationMode=NoTorque  RzMotionActuationMode=ComputedMotion  RzSensePosition=off  RzSenseVelocity=off  RzSenseAcceleration=off  RzSenseTorqueForce=off  RzSenseLowerLimitTorqueForce=off  RzSenseUpperLimitTorqueForce=off
  Gimbal Watts Upper Body : sm_lib/Joints/Gimbal Joint  JointMode=Normal  CompositeWrenchDir=FollowerOnBase  CompositeWrenchFrame=BaseFrame  SenseConstraintForce=off  SenseConstraintTorque=off  SenseTotalForce=off  SenseTotalTorque=off  RxPositionTargetSpecify=off  RxPositionTargetPriority=High  RxPositionTargetValue=0  RxPositionTargetValueUnits=deg  RxVelocityTargetSpecify=off  RxVelocityTargetPriority=High  RxVelocityTargetValue=0  RxVelocityTargetValueUnits=deg/s  RxEquilibriumPosition=0  RxEquilibriumPositionUnits=deg  RxSpringStiffness=0  RxSpringStiffnessUnits=N*m/deg  RxDampingCoefficient=0  RxDampingCoefficientUnits=N*m/(deg/s)  RxLowerLimitSpecify=off  RxLowerLimitBound=-90  RxLowerLimitBoundUnits=deg  RxLowerLimitStiffness=1e4  RxLowerLimitStiffnessUnits=N*m/deg  RxLowerLimitDamping=10  RxLowerLimitDampingUnits=N*m/(deg/s)  RxLowerLimitTransitionRegionWidth=0.1  RxLowerLimitTransitionRegionWidthUnits=deg  RxUpperLimitSpecify=off  RxUpperLimitBound=90  RxUpperLimitBoundUnits=deg  RxUpperLimitStiffness=1e4  RxUpperLimitStiffnessUnits=N*m/deg  RxUpperLimitDamping=10  RxUpperLimitDampingUnits=N*m/(deg/s)  RxUpperLimitTransitionRegionWidth=0.1  RxUpperLimitTransitionRegionWidthUnits=deg  RxTorqueActuationMode=NoTorque  RxMotionActuationMode=ComputedMotion  RxSensePosition=off  RxSenseVelocity=off  RxSenseAcceleration=off  RxSenseTorqueForce=off  RxSenseLowerLimitTorqueForce=off  RxSenseUpperLimitTorqueForce=off  RyPositionTargetSpecify=off  RyPositionTargetPriority=High  RyPositionTargetValue=0  RyPositionTargetValueUnits=deg  RyVelocityTargetSpecify=off  RyVelocityTargetPriority=High  RyVelocityTargetValue=0  RyVelocityTargetValueUnits=deg/s  RyEquilibriumPosition=0  RyEquilibriumPositionUnits=deg  RySpringStiffness=0  RySpringStiffnessUnits=N*m/deg  RyDampingCoefficient=0  RyDampingCoefficientUnits=N*m/(deg/s)  RyLowerLimitSpecify=off  RyLowerLimitBound=-90  RyLowerLimitBoundUnits=deg  RyLowerLimitStiffness=1e4  RyLowerLimitStiffnessUnits=N*m/deg  RyLowerLimitDamping=10  RyLowerLimitDampingUnits=N*m/(deg/s)  RyLowerLimitTransitionRegionWidth=0.1  RyLowerLimitTransitionRegionWidthUnits=deg  RyUpperLimitSpecify=off  RyUpperLimitBound=90  RyUpperLimitBoundUnits=deg  RyUpperLimitStiffness=1e4  RyUpperLimitStiffnessUnits=N*m/deg  RyUpperLimitDamping=10  RyUpperLimitDampingUnits=N*m/(deg/s)  RyUpperLimitTransitionRegionWidth=0.1  RyUpperLimitTransitionRegionWidthUnits=deg  RyTorqueActuationMode=NoTorque  RyMotionActuationMode=ComputedMotion  RySensePosition=off  RySenseVelocity=off  RySenseAcceleration=off  RySenseTorqueForce=off  RySenseLowerLimitTorqueForce=off  RySenseUpperLimitTorqueForce=off  RzPositionTargetSpecify=off  RzPositionTargetPriority=High  RzPositionTargetValue=0  RzPositionTargetValueUnits=deg  RzVelocityTargetSpecify=off  RzVelocityTargetPriority=High  RzVelocityTargetValue=0  RzVelocityTargetValueUnits=deg/s  RzEquilibriumPosition=0  RzEquilibriumPositionUnits=deg  RzSpringStiffness=0  RzSpringStiffnessUnits=N*m/deg  RzDampingCoefficient=0  RzDampingCoefficientUnits=N*m/(deg/s)  RzLowerLimitSpecify=off  RzLowerLimitBound=-90  RzLowerLimitBoundUnits=deg  RzLowerLimitStiffness=1e4  RzLowerLimitStiffnessUnits=N*m/deg  RzLowerLimitDamping=10  RzLowerLimitDampingUnits=N*m/(deg/s)  RzLowerLimitTransitionRegionWidth=0.1  RzLowerLimitTransitionRegionWidthUnits=deg  RzUpperLimitSpecify=off  RzUpperLimitBound=90  RzUpperLimitBoundUnits=deg  RzUpperLimitStiffness=1e4  RzUpperLimitStiffnessUnits=N*m/deg  RzUpperLimitDamping=10  RzUpperLimitDampingUnits=N*m/(deg/s)  RzUpperLimitTransitionRegionWidth=0.1  RzUpperLimitTransitionRegionWidthUnits=deg  RzTorqueActuationMode=NoTorque  RzMotionActuationMode=ComputedMotion  RzSensePosition=off  RzSenseVelocity=off  RzSenseAcceleration=off  RzSenseTorqueForce=off  RzSenseLowerLimitTorqueForce=off  RzSenseUpperLimitTorqueForce=off
  Pin Slot Watts Pivot : Subsystem
      mask Display: image('sm_car_pinslot_joint_IMAGE.png');
  Universal Pivot Upper : Subsystem
      mask Display: image('sm_car_universal_icon.png');
  Universal Watts Pivot Lower : Subsystem
      mask Display: image('sm_car_universal_icon.png');
  Watts Link Lower : $bdroot/Rod  VariantControl=Steer  popup_leftRight=Left  hp_in=hp_wattsl_body  hp_out=hp_wattsl_pivot  rod_mass=wattsl_mass  clr_conn_rod=clr_conn_rod  opc_conn_rod=opc_conn_rod  size_conn_rod=size_conn_rod  clr_rod=clr_link  opc_rod=opc_link  radius_rod=radius_link
  Watts Link Pivot : Subsystem  VariantControl=Steer  mask{popup_leftRight=Left, hp_b=hp_wattsu_pivot, hp_f=hp_wattsl_pivot, hp_piv=hp_wattsp_axle, rod_mass=wattsp_mass, clr_conn_rod=clr_conn_rod, opc_conn_rod=opc_conn_rod, size_conn_rod=size_conn_rod, clr_rod=clr_link, opc_rod=opc_link, radius_rod=radius_link}
      mask prompts: popup_leftRight "Left/Right"; hp_b "HP B [xyz] (m)"; hp_f "HP F [xyz] (m)"; hp_piv "HP Pivot [xyz] (m)"; rod_mass "Mass (kg)"
      mask init:
      | if(popup_leftRight == 1)
      |     rhs_rod = 1;
      | elseif(popup_leftRight == 2)
      |     rhs_rod = -1;
      | end
      mask TypeOptions popup_leftRight: Left | Right
      mask TypeOptions clr_conn_rod:
      | Vis
      | HP A/GraphicDiffuseColor | Vis
      | HP F/GraphicDiffuseColor
      mask TypeOptions opc_conn_rod:
      | Vis
      | HP A/GraphicOpacity | Vis
      | HP F/GraphicOpacity
      mask TypeOptions clr_rod: Rod BP/clr_solid | Rod PF/clr_solid
      mask TypeOptions opc_rod: Rod BP/opc_solid | Rod PF/opc_solid
      mask TypeOptions radius_rod: Rod BP/rad_solid | Rod PF/rad_solid
      mask DialogControl cont_rod Prompt: Rod
      mask DialogControl grp_rod Prompt: Rod
      mask DialogControl cont_vis_rod Prompt: Visualization
      mask DialogControl text_clr_rod Prompt: Color [RGB]
      mask DialogControl text_opc_rod Prompt: Opac. (0-1)
      mask DialogControl text_size_rod Prompt: Size (m)
      mask DialogControl text_conn_rod Prompt: Connections
      mask DialogControl text_rod_rod Prompt: Rod
      mask Display: image('sm_car_vehicle_linkage_link_IMAGE.png');
  Watts Link Upper : $bdroot/Rod  VariantControl=Steer  popup_leftRight=Left  hp_in=hp_wattsu_body  hp_out=hp_wattsu_pivot  rod_mass=wattsu_mass  clr_conn_rod=clr_conn_rod  opc_conn_rod=opc_conn_rod  size_conn_rod=size_conn_rod  clr_rod=clr_link  opc_rod=opc_link  radius_rod=radius_link
  WU : PMIOPort  Side=Left
  WL : PMIOPort  Port=2  Side=Left
  WP : PMIOPort  Port=3  Side=Right
  connections:
  Pin Slot Watts Pivot/RConn1 -- Watts Link Pivot/RConn2
  "Gimbal Watts Lower Body "/LConn1 -- Watts Link Lower/RConn1
  Universal Watts Pivot Lower/LConn1 -- Watts Link Pivot/LConn1
  Universal Pivot Upper/LConn1 -- Watts Link Pivot/RConn1
  Gimbal Watts Upper Body/LConn1 -- WU/RConn1
  Pin Slot Watts Pivot/LConn1 -- WP/RConn1
  "Gimbal Watts Lower Body "/RConn1 -- WL/RConn1
  Watts Link Lower/LConn1 -- Universal Watts Pivot Lower/RConn1
  Universal Pivot Upper/RConn1 -- Watts Link Upper/LConn1
  Gimbal Watts Upper Body/RConn1 -- Watts Link Upper/RConn1

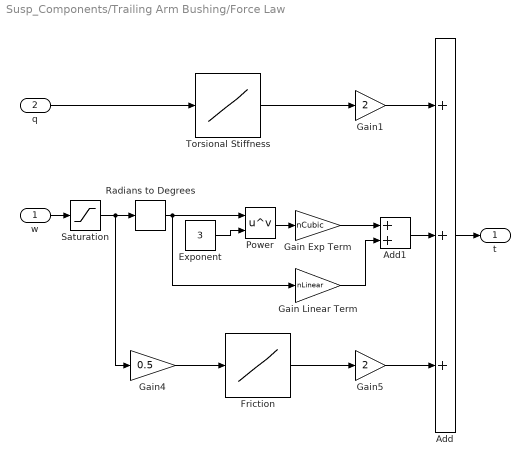
== system Susp_Components/Trailing Arm Bushing/Force Law ==
  w : Inport
  q : Inport  Port=2
  Add : Sum  Inputs=+++
  Add1 : Sum
  Exponent : Constant  Value=3
  Friction : Lookup_n-D  NumberOfTableDimensions=1  BreakpointsForDimension1=wFriction  Table=trqFriction  InterpMethod=Cubic spline  InternalRulePriority=Speed  RndMeth=Simplest
  Gain Exp Term : Gain  Gain=nCubic
  Gain Linear Term : Gain  Gain=nLinear
  Gain1 : Gain  Gain=2
  Gain4 : Gain  Gain=0.5
  Gain5 : Gain  Gain=2
  Power : Math  Operator=pow
  Radians to Degrees : simulink_extras/Transformations/Radians to Degrees
  Saturation : Saturate  UpperLimit=0.1  LowerLimit=-0.1
  Torsional Stiffness : Lookup_n-D  NumberOfTableDimensions=1  BreakpointsForDimension1=qStiffness  Table=trqStiffness  InterpMethod=Cubic spline  InternalRulePriority=Speed  RndMeth=Simplest
  t : Outport
  wires:
  Add/1 -> t/1
  q/1 -> Torsional Stiffness/1
  Exponent/1 -> Power/2
  Gain5/1 -> Add/3
  Gain1/1 -> Add/1
  Radians to Degrees/1 -> Gain Linear Term/1, Power/1
  w/1 -> Saturation/1
  Add1/1 -> Add/2
  Torsional Stiffness/1 -> Gain1/1
  Power/1 -> Gain Exp Term/1
  Friction/1 -> Gain5/1
  Gain4/1 -> Friction/1
  Gain Exp Term/1 -> Add1/1
  Saturation/1 -> Gain4/1, Radians to Degrees/1
  Gain Linear Term/1 -> Add1/2
